simulink model "BouncingBall"  (R2021a)
settings: Solver=VariableStepAuto  StartTime=0.0  StopTime=10  RelTol=1e-3
undefined symbols (not defined in the file): b, k, r
libraries: vrlib x2
settings Model: Creator=Alvan  LastModifiedBy=Alvan

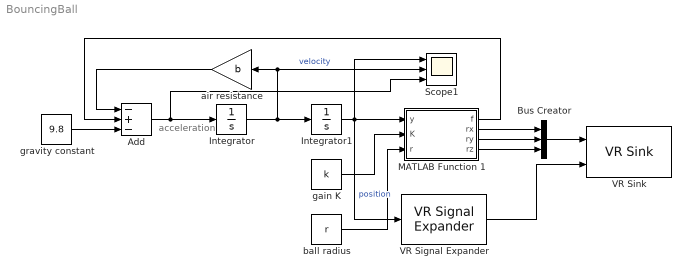
== system BouncingBall ==
  note: acceleration
  Add : Sum  Inputs=-+-
  Bus Creator : BusCreator  Inputs=3
  Integrator : Integrator
  Integrator1 : Integrator  InitialCondition=20
  MATLAB Function 1 : MATLAB Function  TreatAsAtomicUnit=on
  Scope1 : Scope  NumInputPorts=3
  VR Signal Expander : vrlib/VR Signal Expander  outwidth=3  outidx=[2]
  VR Sink : vrlib/VR Sink  InstantiateOnLoad=on  SampleTime=0.1  ViewEnable=on  RemoteChange=off  RemoteView=off  FieldsWritten=Bola.scale.3.1.1.double#Bola.translation.3.1.1.double  WorldFileName=3dBolaPantul.x3d  AutoView=off  VideoDimensions=[]  AllowVariableSize=off
  air resistance : Gain  Gain=b
  "ball radius " : Constant  Value=r
  gain K : Constant  Value=k
  gravity constant : Constant  Value=9.8
  wires:
  MATLAB Function 1/2(rx) -> Bus Creator/1
  "ball radius "/1 -> MATLAB Function 1/3(r)
  MATLAB Function 1/1(f) -> Add/2
  gain K/1 -> MATLAB Function 1/2(K)
  MATLAB Function 1/4(rz) -> Bus Creator/3
  air resistance/1 -> Add/1
  Add/1 -> Scope1/3, Integrator/1
  Integrator/1 -> Scope1/2, air resistance/1, Integrator1/1  "velocity"
  Integrator1/1 -> Scope1/1, VR Signal Expander/1, MATLAB Function 1/1(y)  "position"
  gravity constant/1 -> Add/3
  MATLAB Function 1/3(ry) -> Bus Creator/2
  Bus Creator/1 -> VR Sink/1
  VR Signal Expander/1 -> VR Sink/2

== matlab function BouncingBall/MATLAB Function 1 ==
  data: y input; f output; K input; r input; rx output; ry output; rz output
function [f, rx, ry, rz] = fcn(y, K, r)
% f adalah reaksi lantai (gaya). Kompresi bola menghasilkan gaya tolak dari
% lantai yang sama dengan komprei ola
% K adalah konstanta
% r adalah jari-jari bola dalam meter

%Menghindari pembagian dengan nol
if(y < 1e-4)
    y = 1e-4;
end

if(y >= r)  % Before collision with the ground
    f = 0
    rx = r;
    ry = r;
    rz = r;
else        % After collision with the ground
    
    f = K*(r-y)

    rx = sqrt(r^3/y);
    ry = y;
    rz = rx;

end
